simulink model "AirRefueling_Platform_IBVS"  (R2022b)
settings: Solver=ode4  StartTime=0.0  StopTime=60  FixedStep=0.01  RelTol=1e-5  AbsTol=1e-4  EnableMultiTasking=on
InitFcn:
  | F16_Init
values from neighbouring files (symbols this model uses):
  airSpeed = 393.72    [F16_Init.m]
  alpha0 = trimAlpha*180/pi    (= 6.62393794015)    [F16_Init.m]
  altitude = 9843    [F16_Init.m]
  b_ref = 30.0    (= 30)    [F16_Init.m]
  C2m = [C(1,:) ... (first row only)    [F16_Init.m]
  Cdr_ = 0.8    [hose_parameter4dock.mat]
  d_f_rc = [4.45;0;-3.81]    [F16_Init.m]
  d_pr_cam = d_pr_rc - d_cam_rc    [F16_Init.m]
  d_pr_rc = [8.2;0.45;-3.3]    [F16_Init.m]
  dLEF = 0    [F16_Init.m]
  dtheta10 = [0 0 0 0 0 0 0 0 0 0]    [hose_parameter4dock.mat]
  dtheta20 = [0 0 0 0 0 0 0 0 0 0]    [hose_parameter4dock.mat]
  fi_flag = 1    [F16_Init.m]
  height = 3000    [hose_parameter4dock.mat]
  k_reel = 0.5    [hose_parameter4dock.mat]
  Kc = [ ... (first row only)    [F16_Init.m]
  kd = 500    [hose_parameter4dock.mat]
  Ki = zeros(4,3)    [F16_Init.m]
  Kp = zeros(4,18)    [F16_Init.m]
  l0 = 1.44444444444    [hose_parameter4dock.mat]
  l1 = 2    [hose_parameter4dock.mat]
  l_density = 4.1    [hose_parameter4dock.mat]
  m0 = 5.92222222222    [hose_parameter4dock.mat]
  mass = 636.94    [F16_Init.m]
  Mdr = 29.5    [hose_parameter4dock.mat]
  N = 10    [hose_parameter4dock.mat]
  p0_rc = [-30.7;1;10]    [F16_Init.m]
  Rdr = 0.305    [hose_parameter4dock.mat]
  Rl = 0.0336    [hose_parameter4dock.mat]
  T_reel_initial = 1610    [hose_parameter4dock.mat]
  theta10 = [0.459903280115 0.432776206681 0.412025416789 0.390288667864 0.365355881715 0.340009787283 0.310854701374 0.281345523746 0.248396428993 0.214590627751]    [hose_parameter4dock.mat]
  theta20 = [0 0 0 0 0 0 0 0 0 0]    [hose_parameter4dock.mat]
  trim_ail = 0.00874607850103852    (= 0.00874607850104)    [F16_Init.m]
  trim_control = [trim_thrust;trim_ele;trim_ail;trim_rud]    [F16_Init.m]
  trim_ele = -2.97973164860638    (= -2.97973164861)    [F16_Init.m]
  trim_rud = 0.0680302158182712    (= 0.0680302158183)    [F16_Init.m]
  trim_state1 = [trim_state;0;0;0;0;0;0]    [F16_Init.m]
  trim_thrust = 2279.08519954656    (= 2279.08519955)    [F16_Init.m]
  visual_err = [0;0;0]    [F16_Init.m]
  vt0 = [120 0 0]    [hose_parameter4dock.mat]
undefined symbols (not defined in the file or in its folder): F, MIL, STD
libraries: etargetslib x11, dspnetwork x10, aerolibconvert2 x4, aerolibasang x4, simulink x2, aerolibatmos2 x2, aerolibwind2 x2, aerolibobsolete x2, aerolibadyn x1, aerolibanimutils x1, slrealtimeiplib x1
(part 3 of 3)

== matlab function AirRefueling_Platform_IBVS/Hose-drogue system/DRdynamics/Hose-Drogue1/Calculate the Orientation of the Links1/MATLAB Function4 ==
  data: a input; a0 input; nd1 input; nd2 input; dn input; dnd1 input; dnd2 input; dtheta1 input; dtheta2 input; l1 input size=1; dl1 input; ddtheta1 output; ddtheta2 output; N parameter; l0 parameter
function [ddtheta1,ddtheta2] = fcn(a,a0,nd1,nd2,dn,dnd1,dnd2,dtheta1,dtheta2,l1,dl1, N, l0)
% theta1,theta2 向量N*1
% omiga,alpha是加油机坐标系的旋转角速度和叫加速度
% a是各节点的加速度
% a0为加油机加速度
% l,dl,ddl是连杆的长度及其一二阶导数

ddtheta1 = zeros(1,N);
ddtheta2 = zeros(1,N);

ddtheta1(1) = nd1(:,1)'*(-(a(:,1)-a0)-2*dl1*dn(:,1)-...
              l1*(dnd1(:,1)*dtheta1(1)+dnd2(:,1)*dtheta2(1)))...
              /(l1*norm(nd1(:,1)));
ddtheta2(1) = nd2(:,1)'*(-(a(:,1)-a0)-2*dl1*dn(:,1)-...
              l1*(dnd1(:,1)*dtheta1(1)+dnd2(:,1)*dtheta2(1)))...
              /(l1*norm(nd2(:,1)));
for i = 2:N
    ddtheta1(i) = nd1(:,i)'*(-(a(:,i)-a(:,i-1))-...
                  l0*(dnd1(:,i)*dtheta1(i)+dnd2(:,i)*dtheta2(i)))...
                  /(l0*norm(nd1(:,i)));
    ddtheta2(i) = nd2(:,i)'*(-(a(:,i)-a(:,i-1))-...
                  l0*(dnd1(:,i)*dtheta1(i)+dnd2(:,i)*dtheta2(i)))...
                  /(l0*norm(nd2(:,i)));
end

== matlab function AirRefueling_Platform_IBVS/Hose-drogue system/DRdynamics/Hose-Drogue1/Calculate the Orientation of the Links1/MATLAB Function5 ==
  data: v0 input; n input; dn input; l1 input; dl1 input; w input; vr output; p0 input; p output; N parameter; l0 parameter; pdr output
function [vr,p,pdr] = fcn(v0,n,dn,l1,dl1,w,p0, N, l0)

% v0为加油机速度
% l,dl是连杆的长度及其一阶导数
% wt为合成风在每个节点的风速
% p0为预留，在计算相对地面的位置时用到

vr = zeros(3,N);
vr(:,1) = v0 - dl1*n(:,1) - l1*dn(:,1) ;
for i = 2:N
    vr(:,i) = vr(:,i-1) - l0*dn(:,i);
end
vr = vr - w;

p = zeros(3,N);
p(:,1) = [0;0;0] - l1*n(:,1);
for i = 2:N
    p(:,i) = p(:,i-1) - l0*n(:,i);
end
pdr = p(:,N) + [-0.3;0;0];
% pdr = p(:,N);

== matlab function AirRefueling_Platform_IBVS/Hose-drogue system/DRdynamics/Hose-Drogue1/MATLAB Function3 ==
  data: n input; alpha output; N parameter
function alpha = fcn(n, N)
% 计算两杆之间的弯折角度，用来粗略的验证恢复力的效果
alpha = zeros(1,N);
for i = 2:N
    mid = n(:,i-1)'*n(:,i);
    if abs(mid) > 1
        mid = mid/abs(mid);
    end
    alpha(i) = acos(mid)/pi*180;
end

== matlab function AirRefueling_Platform_IBVS/Receiver System/Guidance ==
  settings: updateMethod=DISCRETE
  data: dd input; estimate_dr2pr input; y output; t input; d_x output; t_d output
function [y,d_x,t_d] = fcn(dd,estimate_dr2pr,t)
%#codegen
%dd是锥管前端位置，dx是锥套位置（dx输入前第三分量换号，已由x,y,h转化为x,y,z）
%dx输入前减去常数：控制中控制的是受油机质心而非锥管前端，所以参考轨迹也要由锥管的参考轨迹转化为受油机质心的参考轨迹。
%控制的目的就是最终令dd和dx相等，让受油机质心跟踪参考位置

% y=dx; 输出y的意思是让受油机飞行的三维距离，和之前初始化定义受油机三维位置不同
%% 理想的对接点是  [9.5100;-1.4550;-0.0830]+[0.2;0;0] 9.5m时是第一节探头进锥套 最多再多0.2m此时是第一节抵住中间小黑圈
persistent aa;
if(isempty(aa))   %%aa(1:3)为锥套平衡位置,(4:6)为锥套实际位置或其滤波位置，(7:9)是锥管实际位置或其滤波位置；
    aa=zeros(9,1);
end

% 这个tt是用来对总体的时间逻辑进行控制的
persistent tt;
if(isempty(tt))
    tt=0;
end
% 这个t_dock是用来记录对接成功的初始时间的，这样就能
persistent t_dock;
if(isempty(t_dock))
    t_dock=0;
end
t_d=t_dock;

% 这个t_lock是用来锁定对接时间的，标识为1时说明已经锁定了对接时间
persistent t_lock;
if(isempty(t_lock))
    t_lock=0;
end

% 判断是否可以脱离对接，再进行下一次的对接
persistent flag_can_dock;
if(isempty(flag_can_dock))
    flag_can_dock=1;
end

persistent nn;    %%nn为前馈量
if(isempty(nn))
    nn=[0;0;0];
end

persistent dx;     %%锥套位置距离其平衡位置的偏差
if(isempty(dx))
    dx=[0;0;0];
end
d_x=dx;

% 使用额外飞行的距离来对碰撞模块和HDU进行验证
extra_flight=[0.5;0;0];
%% y为期望轨迹
%30s之前都是固定期望轨迹飞行；24s之后更新dx，并进行滤波（因为dx是0，所以要提前几秒开始滤波）；30s之后根据迭代学习前馈进行飞行；
% tt是上次对接成功时候记录的时间
t1=t-tt;
if t1<20
    y=[8;-1.8;0.4];
    aa(1:3)=y;
elseif t1<30
    y = aa(1:3);
    if t1>24 && t1<25
        % 此时的aa(1:3)约等于[8;-1.8;0.4]，estimate_pr2dt=[1.61;0.345;-0.483]
        dx = aa(1:3)+ estimate_dr2pr;
    end
    if t1>25
        dx(1:3) = 3/4 * dx(1:3) + 1/4 * (aa(1:3) + estimate_dr2pr);
    end
else   
    y = [dx(1)+nn(1);dx(2)+nn(2);dx(3)+nn(3)]+extra_flight ; 
%     y = 0.5 * ([dx(1)+nn(1);dx(2)+nn(2);dx(3)+nn(3)]+[dx(1)+dd(1);dx(2)+dd(2);dx(3)+dd(3)]);     
%%  这里是近距离对接过程的判断
    if abs(dd(1)-dx(1))<0.01 && flag_can_dock == 1  % 状态为可以对接 且 锥管锥套距离达到对接要求 认为是一次对接
       % 认为已经对接上了 所以标志位要清零, 同时记录对接的时间t_dock
       flag_can_dock = 0;
       t_lock = 1;
       if(t_lock == 1 && flag_can_dock == 0)
           % 在对接成功时，虽然满足0.01的条件，但是不满足后面==1的条件 所以对接时间不会多次记录
          t_dock = t;
       end
    end
    
   % t_dock保存的就是对接成功的时间 当保持的时间大于20s时，才进行下一次对接
   % 在对接状态 且 持续时间超过了10s 就设置为脱离状态
   if(t-t_dock>=10 && flag_can_dock == 0 )
       flag_can_dock=1;
           % 如果对接的时间到 那么锥套椎管放开接触 标志位置1，意味着可以对接
       if(flag_can_dock == 1)
           % 更新前馈量 aa(4:6)存储的是锥套的滤波位置 aa(7:9)存储的是椎管的滤波位置
           nn=nn+[0.6*sat((aa(4)-aa(7))/0.6);0.6*sat((aa(5)-aa(8))/0.6);0.6*sat((aa(6)-aa(9))/0.6)];

           % 省去了前面的过程  时间如果一减掉 调用脚本的时候就跳出这个代码范围 相当于回到第10s时候的状态
           tt=t-10;
       end   
   end    
          
    % 当距离小于0.4m的时候，进行滤波
    if abs(dd(1)-dx(1))<0.4 && flag_can_dock == 1
        aa(4:6)=2/3 * aa(4:6)+ 1/3 * dx;
        aa(7:9)=2/3 * aa(7:9)+ 1/3 * dd;
    end  
    % 当小于0.5m大于0.4m的时候，记录位置
    if abs(dd(1)-dx(1))<0.5 && flag_can_dock == 1
        aa(4:6)=dx;
        aa(7:9)=dd;
    end 
end

== matlab function AirRefueling_Platform_IBVS/Visual process/VehicleDataParse ==
  data: Data input; CopterID output; Length input; Out output; checksum input; len input
function [CopterID,Out] = fcn(Data,Length,checksum,len)

% 设定静态变量，在数据校验失败时，保持上一时刻值
persistent DataOut;
if isempty(DataOut)
    DataOut=zeros(16,1);
end
persistent cpID;
if isempty(cpID)
    cpID=0;
end

% 如果包长不等于设定值，这个包丢弃，使用原来的值
if Length ~= len %如果包长度不匹配，校验不通过，那么使用上一时刻值
    Out=DataOut;
    CopterID=cpID;
    return;
end

CkSum = typecast(Data(1:4), 'int32');
if CkSum ~= checksum %如果校验码不匹配，校验不通过，那么使用上一时刻值
    Out=DataOut;
    CopterID=cpID;
    return;    
end

% 提取数据
CpIDTmp = typecast(Data(5:8), 'int32');
DataTmp = typecast(Data(9:136), 'double');
% DataTmp=zeros(16,1);
for i=1:16
    idx = (i-1)*8+9;
    DataTmp(i) = typecast(Data(idx:idx+7), 'double');
end



% 配置输出数据
CopterID = double(CpIDTmp);
Out = DataTmp;

% 记录上一时刻值
cpID=CopterID;
DataOut=Out;

== matlab function AirRefueling_Platform_IBVS/Hose-drogue system/DRdynamics/Hose-Drogue1/Calculate the Acceleration of the Links1/MATLAB Function ==
  data: n input; m1 input; T output; m0 parameter; N parameter
function T = fcn(n,m1, m0,N)

% n = 连杆的方向向量，想上为正 向量3*N
% m = 连杆的质量 向量1*N

%%%%求张力t%%%%%%%%%%%%%%%%%%%%%%%%%%%%%%%%%%%%%%%%%%%%%%%%%%%%%%
T = zeros(N,N);

T(1,1) = 1;
T(1,2) = - n(:,1)'*n(:,2);
T(N,N-1) = -1/m0*n(:,N-1)'*n(:,N);
T(N,N) = 1/m0 + 1/m0;             %注意这里很重要！！

T(2,1) = -1/m1*n(:,1)'*n(:,2);
T(2,2) = 1/m1 + 1/m0;
T(2,3) = -1/m0*n(:,2)'*n(:,3);

for i = 3:N-1
    T(i,i-1) = -1/m0*n(:,i-1)'*n(:,i);
    T(i,i) = 1/m0 + 1/m0;
    T(i,i+1) = -1/m0*n(:,i)'*n(:,i+1);
end

== matlab function AirRefueling_Platform_IBVS/Tanker system/  ==
  data: u input; y output

function y = WindTurFromTank(u)
%#codegen

%横纵向气流角速度等下计算长度
c_lat=4;
c_lon=4;

%两端参考点
u1 = u+[0 ,c_lat ,0]';
u2 = u+[0 ,-c_lat, 0]';

yy1 = TankerVortexWindField(u1);
yy2 = TankerVortexWindField(u2);

%计算x轴向滚转角速度
yp = (yy1(3) - yy2(3))/4/c_lat;

u3=u+[c_lon, 0,0]';
u4=u+[-c_lon ,0,0]';
yy3 = TankerVortexWindField(u3);
yy4 = TankerVortexWindField(u4);

%俯仰角速度计算
yq = -(yy3(3) - yy4(3))/4/c_lon;

%偏航角速度设为0
yr = 0;

%质心处风场计算
y_uvw = TankerVortexWindField(u);


%y = [y_uvw(1);y_uvw(2);y_uvw(3);-yp;-yq;-yr]*0.5;
y = [y_uvw(1);y_uvw(2);y_uvw(3);-yp;-yq;-yr];

== matlab function AirRefueling_Platform_IBVS/Hose-drogue system/DRdynamics/HDU/MATLAB Function1 ==
  data: l1 input; l1initial input; dl1 input; flag1 output size=1; l1out output; dl1out output; ddl1 input; ddl1out output
function [flag1,l1out,dl1out,ddl1out] = fcn(l1,l1initial,dl1,ddl1)
% 如果第一根管子的长度比初始值大 或者 第一根管子的加速度>0 那么就是要控制了 flag从0变1开始积分
if (l1 > l1initial) || (l1 == l1initial && dl1 > 0)
    flag1 = 1;
    l1out = l1initial;
    dl1out = 0;
    ddl1out = 0;
else
    flag1 = 0;
    l1out = l1;
    dl1out = dl1;
    ddl1out = ddl1;
end

== matlab function AirRefueling_Platform_IBVS/Hose-drogue system/Bow Wave Effect/Bow Wave Effect Function ==
  data: x input; Fx output; y input; z input; Fy output; Fz output
function [Fx,Fy,Fz] = F_rc2dr(x,y,z)
Cx1 = 91.6170;
Cx2 = 0.3220;
Cx3 = 3.8870;
Cx4 = 2.7359;
Cx5 = 2.4939;
Cx6 = 309.7709;
Cx7 = 0.3237;
Cx8 = 0.3851;
Cx9 = 1.1471;

Cy1 = 223.3210;
Cy2 = 0.2082;
Cy3 = 0.8102;
Cy4 = 0.6555;

Cz1 = 173.2021;
Cz2 = 0.2141;
Cz3 = 0.5697;
Cz4 = 0.7038;

if x > 5.6493
    Fx = 0;
elseif x > 3.0893
    Fx = Cx1*(1-Cx2*(x-Cx3)^2)*exp(-y^2/Cx4)*exp(z/Cx5);
else
    Fx = Cx1*(1-Cx2*(x-Cx3)^2)*exp(-y^2/Cx4)*exp(z/Cx5)...
       + Cx6*(1-Cx7*x)*exp(-y^2/Cx8)*exp(z/Cx9);
end

if x > 4.8031
    Fy = 0;
else
    Fy = Cy1*(1-Cy2*x)*(y*exp(-y^2/Cy3))*exp(z/Cy4);
end

if x > 4.6275
    Fz = 0;
else
    Fz = -Cz1*(1-Cz2*x)*exp(-y^2/Cz3)*exp(z/Cz4);
end

== matlab function AirRefueling_Platform_IBVS/Hose-drogue system/Total Turbulence   ==
  data: u1 input; u input; y output
function y = Dr_wind2Frc(u1,u)
%#codegen

Ve=120;
rho = 0.98;
Q=0.5*rho*Ve^2;
S=0.38;
CD=0.81*0.8;

uu=u(1);
vv=u(2);
ww=u(3);

%beta = acos(sqrt(vv^2+ww^2)/abs(uu));
%theta = atan(ww/vv);

C_beta = 0.3979;

yx=rho*S*CD*Ve*uu;
yy=Q*S*C_beta*vv/Ve;
yz=Q*S*C_beta*ww/Ve;

% 这个y_v是有涡流+自然风所得到的速度换算成的位置偏移
y_v = [yx,yy,yz]';
y=[y_v;u1+y_v];

== matlab function AirRefueling_Platform_IBVS/Hose-drogue system/DRdynamics/HDU/MATLAB Function2 ==
  data: l_1 input; T0 input; Tt output size=1; t input; dl input; l1 parameter; k_reel parameter; kd parameter
function Tt = fcn(l_1,T0,t,dl, l1,k_reel,kd)
Treel = T0*(l_1/l1)^k_reel;
Tt = t - Treel - kd*dl;

== matlab function AirRefueling_Platform_IBVS/Receiver System/F16 Nonlinear Model/Environment Models/mass variable ==
  data: g input; y output; mass input; time input
function y = fcn(g,mass,time)

if(time<50)
    y = mass*g;
else
    y = (mass+(time-50)*2)*g
end
